simulink model "Simulink_5"  (R2016b)
settings: Solver=VariableStepAuto  StartTime=0.0  StopTime=50  RelTol=1e-3
values from neighbouring files (symbols this model uses):
  C_lat = [1 0 0 0 ... (first row only)    [ejercicio07_lateral_C.m]
  D_lat = zeros(2)    [ejercicio07_lateral_C.m]
  dt = 0.001    [ejercicio07_lateral_C.m]    (also in ejercicio07_longitudinal_C.m)
  F_lat = A_lat*Tm + I    [ejercicio07_lateral_C.m]
  G_lat = B_lat*Tm    [ejercicio07_lateral_C.m]
  Kc = Kc_a(:,1:4)    [ejercicio07_lateral_C.m]    (also in ejercicio07_longitudinal_C.m)
  Ki = -Kc_a(:,5:6)    [ejercicio07_lateral_C.m]    (also in ejercicio07_longitudinal_C.m)
  Ko_d = dlqe(F_lat,G_lat,C_lat,V1,V2)    [ejercicio07_lateral_C.m]    (also in ejercicio07_longitudinal_C.m = dlqe(F_lon,G_lon,C_lon,V1,V2))
  PreC = [Cyr*(I-Fyr)^(-1)*G_lat+D_lat]^(-1)    [ejercicio07_lateral_C.m]    (also in ejercicio07_longitudinal_C.m = [Cyr*(I-Fyr)^(-1)*G_lon+D_lon]^(-1))
  tau_a = 0.5    [ejercicio07_lateral_C.m]
  tau_r = 1/20    (= 0.05)    [ejercicio07_lateral_C.m]
  Tm = 0.003    [ejercicio07_lateral_C.m]    (also in ejercicio07_longitudinal_C.m)
undefined symbols (not defined in the file or in its folder): DiscIntNeverNeededParam, Ko
undefined symbols (not defined in the file): sys_lat
(part 2 of 2)

== system Simulink_5/Ejercicio 5/EJERCICIO 5 DISCRETO/COMPARATIVA/Comparativa modal/Control lateral con observador de estados %bien/Actuadores ==
  u : Inport
  Aleron : Subsystem
  Demux : Demux  Outputs=2
  Mux2 : Mux  Inputs=2
  Scope : Scope
  TIMÓN : Subsystem
  mv : Outport
  wires:
  u/1 -> Demux/1
  Mux2/1 -> mv/1, Scope/1
  Demux/1 -> Aleron/1(u_a)
  Demux/2 -> TIMÓN/1(u_r)
  Aleron/1(delta_a) -> Mux2/1
  TIMÓN/1(delta_r) -> Mux2/2

== system Simulink_5/Ejercicio 5/EJERCICIO 5 DISCRETO/COMPARATIVA/Comparativa modal/Control lateral con observador de estados %bien/Dinamica Lateral ==
  mv : Inport
  Integrator5 : Integrator
  Km1 : Gain  Gain=D  Multiplication=Matrix(K*u)
  Km10 : Gain  Gain=A  Multiplication=Matrix(K*u)
  Km2 : Gain  Gain=C  Multiplication=Matrix(K*u)
  Km8 : Gain  Gain=B  Multiplication=Matrix(K*u)
  Sum1 : Sum  Inputs=++|
  Sum12 : Sum  Inputs=|++
  y : Outport
  wires:
  Km8/1 -> Sum12/1
  Sum12/1 -> Integrator5/1
  Integrator5/1 -> Km10/1, Km2/1  "x"
  Km10/1 -> Sum12/2
  Km2/1 -> Sum1/2
  Km1/1 -> Sum1/1
  Sum1/1 -> y/1
  mv/1 -> Km8/1, Km1/1

== system Simulink_5/Ejercicio 5/EJERCICIO 5 DISCRETO/COMPARATIVA/Comparativa modal/Control lateral con observador de estados %bien/OBSERVADOR1 ==
  u : Inport
  y : Inport  Port=2
  Integrator5 : Integrator
  Km1 : Gain  Gain=D  Multiplication=Matrix(K*u)
  Km10 : Gain  Gain=A  Multiplication=Matrix(K*u)
  Km2 : Gain  Gain=C  Multiplication=Matrix(K*u)
  Km3 : Gain  Gain=Ko  Multiplication=Matrix(K*u)
  Km8 : Gain  Gain=B  Multiplication=Matrix(K*u)
  Sum1 : Sum  Inputs=++|
  Sum12 : Sum  Inputs=+++
  Sum2 : Sum  Inputs=+-|
  xest : Outport
  wires:
  Km8/1 -> Sum12/1
  Sum12/1 -> Integrator5/1
  Integrator5/1 -> Km2/1, Km10/1, xest/1  "xe"
  Km10/1 -> Sum12/3
  Km2/1 -> Sum1/2
  Km1/1 -> Sum1/1
  Sum1/1 -> Sum2/2  "ye"
  u/1 -> Km8/1, Km1/1
  y/1 -> Sum2/1
  Sum2/1 -> Km3/1
  Km3/1 -> Sum12/2

== system Simulink_5/Ejercicio 5/EJERCICIO 5 DISCRETO/COMPARATIVA/Comparativa modal/Control lateral con observador de estados %bien/SENSORES ==
  y : Inport
  Add2 : Sum
  Add3 : Sum
  Demux : Demux  Outputs=2
  Mux2 : Mux  Inputs=2
  Ruido de medida1 : RandomNumber  Variance=1e-6  Seed=123456  SampleTime=dt
  Ruido de medida2 : RandomNumber  Variance=1e-6  Seed=123456  SampleTime=dt
  ym : Outport
  wires:
  y/1 -> Demux/1
  Ruido de medida1/1 -> Add2/1
  Add2/1 -> Mux2/1
  Demux/1 -> Add2/2
  Mux2/1 -> ym/1
  Demux/2 -> Add3/1
  Add3/1 -> Mux2/2
  Ruido de medida2/1 -> Add3/2

== system Simulink_5/Ejercicio 5/EJERCICIO 5 DISCRETO/COMPARATIVA/Comparativa Integral/CONTROL LATERAL DISCRETO ACCION INTEGRAL %bien/Actuadores/Aleron ==
  u_a : Inport
  Transfer Fcn : TransferFcn  Numerator=[1/tau_a]  Denominator=[1 1/tau_a]
  delta_a : Outport
  wires:
  u_a/1 -> Transfer Fcn/1
  Transfer Fcn/1 -> delta_a/1

== system Simulink_5/Ejercicio 5/EJERCICIO 5 DISCRETO/COMPARATIVA/Comparativa Integral/CONTROL LATERAL DISCRETO ACCION INTEGRAL %bien/Actuadores/TIMÓN ==
  u_r : Inport
  Transfer Fcn : TransferFcn  Numerator=[1/tau_r]  Denominator=[1 1/tau_r]
  delta_r : Outport
  wires:
  u_r/1 -> Transfer Fcn/1
  Transfer Fcn/1 -> delta_r/1

== system Simulink_5/Ejercicio 5/EJERCICIO 5 DISCRETO/COMPARATIVA/Comparativa Integral/Control laterall con accion integral %bien/Actuadores/Aleron ==
  u_a : Inport
  Transfer Fcn : TransferFcn  Numerator=[1/tau_a]  Denominator=[1 1/tau_a]
  delta_a : Outport
  wires:
  u_a/1 -> Transfer Fcn/1
  Transfer Fcn/1 -> delta_a/1

== system Simulink_5/Ejercicio 5/EJERCICIO 5 DISCRETO/COMPARATIVA/Comparativa Integral/Control laterall con accion integral %bien/Actuadores/TIMÓN ==
  u_r : Inport
  Transfer Fcn : TransferFcn  Numerator=[1/tau_r]  Denominator=[1 1/tau_r]
  delta_r : Outport
  wires:
  u_r/1 -> Transfer Fcn/1
  Transfer Fcn/1 -> delta_r/1

== system Simulink_5/Ejercicio 5/EJERCICIO 5 DISCRETO/COMPARATIVA/Comparativa modal/CONTROL LATERAL DISCRETO %bien/Actuadores/Aleron ==
  u_a : Inport
  Transfer Fcn : TransferFcn  Numerator=[1/tau_a]  Denominator=[1 1/tau_a]
  delta_a : Outport
  wires:
  u_a/1 -> Transfer Fcn/1
  Transfer Fcn/1 -> delta_a/1

== system Simulink_5/Ejercicio 5/EJERCICIO 5 DISCRETO/COMPARATIVA/Comparativa modal/CONTROL LATERAL DISCRETO %bien/Actuadores/TIMÓN ==
  u_r : Inport
  Transfer Fcn : TransferFcn  Numerator=[1/tau_r]  Denominator=[1 1/tau_r]
  delta_r : Outport
  wires:
  u_r/1 -> Transfer Fcn/1
  Transfer Fcn/1 -> delta_r/1

== system Simulink_5/Ejercicio 5/EJERCICIO 5 DISCRETO/COMPARATIVA/Comparativa modal/Control lateral con observador de estados %bien/Actuadores/Aleron ==
  u_a : Inport
  Transfer Fcn : TransferFcn  Numerator=[1/tau_a]  Denominator=[1 1/tau_a]
  delta_a : Outport
  wires:
  u_a/1 -> Transfer Fcn/1
  Transfer Fcn/1 -> delta_a/1

== system Simulink_5/Ejercicio 5/EJERCICIO 5 DISCRETO/COMPARATIVA/Comparativa modal/Control lateral con observador de estados %bien/Actuadores/TIMÓN ==
  u_r : Inport
  Transfer Fcn : TransferFcn  Numerator=[1/tau_r]  Denominator=[1 1/tau_r]
  delta_r : Outport
  wires:
  u_r/1 -> Transfer Fcn/1
  Transfer Fcn/1 -> delta_r/1

== matlab function Simulink_5/Ejercicio 5/EJERCICIO 5 DISCRETO/CONTROL LATERALDISCRETO FBW/Computador digital/Algoritmo de control ==
  settings: updateMethod=DISCRETE  sampleTime=Tm
  data: Tm input; F input; G input; C input; D input; CO output; Ki input; Kc input; Kod input; sp input; y input size=2; mv input
function CO  = fcn(Tm,F,G,C,D,Ki,Kc,Kod,sp,y,mv)
persistent  int_error xe  
if isempty(int_error)
        int_error = [0 0]';
        xe = [0 0 0 0]';
    
end
%error
error=sp-y;

%accion integral
int_error = int_error + error*Tm;


%observador
ye = C*xe + D*mv;
xe = F*xe +G*mv +Kod*(y-ye);
%señal de control
u= Ki*int_error-Kc*xe;

CO = u;
